simulink subsystem "Piero"  (R2023b)
settings: Solver=VariableStepAuto  StartTime=0.0  StopTime=10.0  RelTol=1e-3
settings Model: Creator=Claudia Ada  LastModifiedBy=pablo

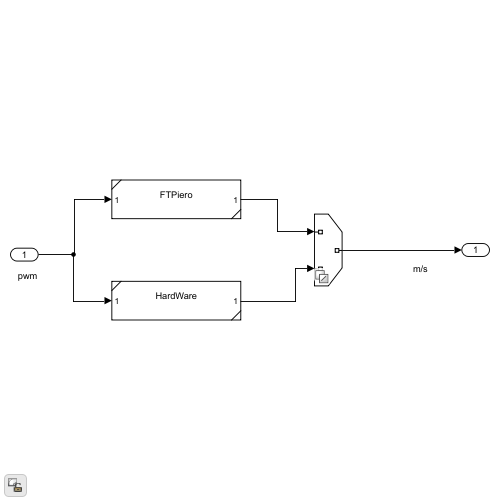
[thumbnail: Simulink's stored preview of the top-level diagram]
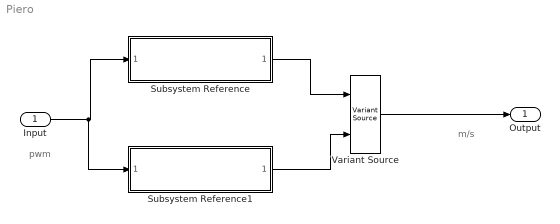
== system Piero ==
  note: m/s
  note: pwm
  Input : Inport  OutDataTypeStr=double
  Subsystem Reference : Subsystem  ReferencedSubsystem=FTPiero
  Subsystem Reference1 : Subsystem  ReferencedSubsystem=HardWare
  Variant Source : VariantSource  VariantControlMode=sim codegen switching
  Output : Outport
  wires:
  Subsystem Reference/1 -> Variant Source/1
  Subsystem Reference1/1 -> Variant Source/2
  Input/1 -> Subsystem Reference1/1, Subsystem Reference/1
  Variant Source/1 -> Output/1
